simulink model "modelo_SEIR"  (R2019b)
settings: Solver=VariableStepAuto  StartTime=0.0  StopTime=360  RelTol=1e-3
undefined symbols (not defined in the file): beta, E0, gamma, I0, R0, S0, sigma
settings Model: Creator=lucia  LastModifiedBy=lucia

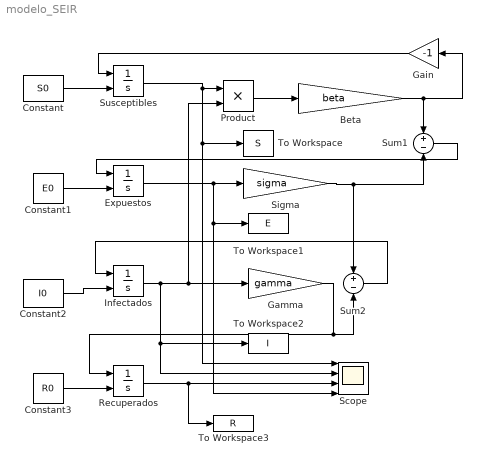
== system modelo_SEIR ==
  Beta : Gain  Gain=beta
  Constant : Constant  Value=S0
  Constant1 : Constant  Value=E0
  Constant2 : Constant  Value=I0
  Constant3 : Constant  Value=R0
  Expuestos : Integrator  InitialConditionSource=external
  Gain : Gain  Gain=-1
  Gamma : Gain  Gain=gamma
  Infectados : Integrator  InitialConditionSource=external
  Product : Product
  Recuperados : Integrator  InitialConditionSource=external
  Scope : Scope  NumInputPorts=4
  Sigma : Gain  Gain=sigma
  Sum1 : Sum  Inputs=+-
  Sum2 : Sum  Inputs=+-
  Susceptibles : Integrator  InitialConditionSource=external
  To Workspace : ToWorkspace  VariableName=S  SaveFormat=Structure With Time  SampleTime=-1
  To Workspace1 : ToWorkspace  VariableName=E  SaveFormat=Structure With Time  SampleTime=-1
  To Workspace2 : ToWorkspace  VariableName=I  SaveFormat=Structure With Time  SampleTime=-1
  To Workspace3 : ToWorkspace  VariableName=R  SaveFormat=Structure With Time  SampleTime=-1
  wires:
  Constant/1 -> Susceptibles/2
  Constant3/1 -> Recuperados/2
  Constant2/1 -> Infectados/2
  Constant1/1 -> Expuestos/2
  Susceptibles/1 -> To Workspace/1, Scope/1, Product/1
  Infectados/1 -> To Workspace2/1, Scope/2, Product/2, Gamma/1
  Product/1 -> Beta/1
  Beta/1 -> Gain/1, Sum1/1
  Expuestos/1 -> To Workspace1/1, Scope/4, Sigma/1
  Sigma/1 -> Sum2/1, Sum1/2
  Sum1/1 -> Expuestos/1
  Sum2/1 -> Infectados/1
  Recuperados/1 -> To Workspace3/1, Scope/3
  Gamma/1 -> Recuperados/1, Sum2/2
  Gain/1 -> Susceptibles/1
